simulink model "shoulder_simulink"  (R2024b)
settings: Solver=VariableStepAuto  StartTime=0.0  StopTime=10  FixedStep=0.02  MaxStep=5e-4  RelTol=1e-3  AbsTol=1e-3  EnableMultiTasking=on
InitFcn:
  | main;
values from neighbouring files (symbols this model uses):
  activ = zeros(35,1)    [main_quat.m]
  fmax = sym('fmax', [length(muscles) 1])    [muscle_derivation.m]
  fmax_optim = x_new(11:11+nmus-1)    [SteadyPosOptEul.m]    (also in SteadyPosOptQuat.m = x_new(qn+1:qn+1+nmus-1); steady_position_optimization.m)
  initCond_optim = [x_new(1:10);zeros(10,1)]    [SteadyPosOptEul.m]
  initEul = params.InitPosOptEul.initCondEul    [main.m]
  initQuat = params.InitPosOptEul.initCondQuat    [main.m]
  lceopt = sym('lceopt', [length(muscles) 1])    [muscle_derivation.m]
  lceopt_optim = x_new(11+nmus:end-1)    [SteadyPosOptEul.m]    (also in SteadyPosOptQuat.m = x_new(qn+1+nmus:end); steady_position_optimization.m = x_new(11+nmus:end))
  lslack = sym('lslack', [length(muscles) 1])    [muscle_derivation.m]
  lslack_optim = lslack_vec    [SteadyPosOptEul.m]    (also in SteadyPosOptQuat.m; steady_position_optimization.m)
  m = [2.0519,0.5464,0.5464,0.525]    [data.m]
  model = das3_readosim(osim_file,[motion_path,'\',mydir '\' musclepoly_file])    [create_motion_files.m]    (also in das3_polynomials.m = das3_readosim(osimfile); data_model_eul.mat = ; data_model_mod.mat = ; main.m = data.params.model)
  params = data.params    [SteadyPosOptEul.m]    (also in data_model.mat = ; main.m)
  s = fx.getSize()    [das3_readosim.m]
undefined symbols (not defined in the file or in its folder): h_ej, initCondOptim, initSimScape, phi_0, r_0, r_10, r_20, r_ej, T_d, X, Y, Z
libraries: sm_lib x80, nesl_utility x39
(part 3 of 3)

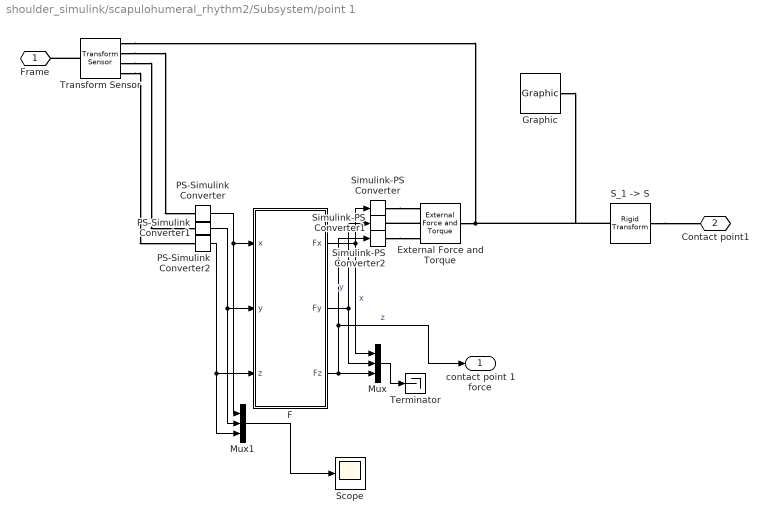
== system shoulder_simulink/scapulohumeral_rhythm2/Subsystem/point 1 ==
  External Force and Torque : sm_lib/Forces and Torques/External Force and Torque  EnableForceX=on  EnableForceY=on  EnableForceZ=on  EnableForce=off  ForceResolutionFrame=World  EnableTorqueX=off  EnableTorqueY=off  EnableTorqueZ=off  EnableTorque=off  TorqueResolutionFrame=AttachedFrame
  F : MATLAB Function  TreatAsAtomicUnit=on
  Graphic : sm_lib/Body Elements/Graphic  GraphicType=Marker  MarkerShape=Sphere  MarkerSize=10  GraphicVisPropType=SimpleVisualProperties  GraphicDiffuseColor=[0 1 0]  GraphicOpacity=1.0  GraphicSpecularColor=[0.5 0.5 0.5 1.0]  GraphicAmbientColor=[0.15 0.15 0.15 1.0]  GraphicEmissiveColor=[0.0 0.0 0.0 1.0]  GraphicShininess=75
  Mux : Mux  Inputs=3
  Mux1 : Mux  Inputs=3
  PS-Simulink Converter : nesl_utility/PS-Simulink Converter  PhysicalDomain=network_engine_domain  SubClassName=ps_output  LeftPortType=input  RightPortType=output  PseudoPeriodic=off  Frequencies=[]  VectorFormat=inherit  Unit=inherit  AffineConversion=off
  PS-Simulink Converter1 : nesl_utility/PS-Simulink Converter  PhysicalDomain=network_engine_domain  SubClassName=ps_output  LeftPortType=input  RightPortType=output  PseudoPeriodic=off  Frequencies=[]  VectorFormat=inherit  Unit=inherit  AffineConversion=off
  PS-Simulink Converter2 : nesl_utility/PS-Simulink Converter  PhysicalDomain=network_engine_domain  SubClassName=ps_output  LeftPortType=input  RightPortType=output  PseudoPeriodic=off  Frequencies=[]  VectorFormat=inherit  Unit=inherit  AffineConversion=off
  "S_1 -> S" : sm_lib/Frames and Transforms/Rigid Transform  RotationMethod=None  FollAlignAxisA=+X  BaseAlignAxisA=+Y  FollAlignAxisB=+Y  BaseAlignAxisB=+Z  RotationStandardAxis=+Z  RotationAngle=0.0  RotationAngleUnits=deg  RotationArbitraryAxis=[0 0 1]  RotationSequenceAxes=FollowerAxes  RotationSequence=XYX  RotationSequenceAngles=[0 0 0]  RotationSequenceAnglesUnits=deg  RotationMatrix=[1 0 0; 0 1 0; 0 0 1]  Quaternion=[1 0 0 0]  TranslationMethod=Cartesian  TranslationCartesianOffset=model.contTS  TranslationCartesianOffsetUnits=m  TranslationStandardAxis=+Z  TranslationStandardOffset=0  TranslationStandardOffsetUnits=m  TranslationROffset=0  TranslationROffsetUnits=m  TranslationThetaOffset=0  TranslationThetaOffsetUnits=deg  TranslationZOffset=0  TranslationZOffsetUnits=m
  Scope : Scope
  Simulink-PS Converter : nesl_utility/Simulink-PS Converter  PhysicalDomain=network_engine_domain  SubClassName=ps_input  LeftPortType=input  RightPortType=output  PseudoPeriodic=off  Frequencies=[]  NoiseDistribution=none  NoiseParameters=[]  Unit=1  AffineConversion=off  FilteringAndDerivatives=provide  SimscapeFilterOrder=1  InputFilterTimeConstant=0.001  UdotUserProvided=0
  Simulink-PS Converter1 : nesl_utility/Simulink-PS Converter  PhysicalDomain=network_engine_domain  SubClassName=ps_input  LeftPortType=input  RightPortType=output  PseudoPeriodic=off  Frequencies=[]  NoiseDistribution=none  NoiseParameters=[]  Unit=1  AffineConversion=off  FilteringAndDerivatives=provide  SimscapeFilterOrder=1  InputFilterTimeConstant=0.001  UdotUserProvided=0
  Simulink-PS Converter2 : nesl_utility/Simulink-PS Converter  PhysicalDomain=network_engine_domain  SubClassName=ps_input  LeftPortType=input  RightPortType=output  PseudoPeriodic=off  Frequencies=[]  NoiseDistribution=none  NoiseParameters=[]  Unit=1  AffineConversion=off  FilteringAndDerivatives=provide  SimscapeFilterOrder=1  InputFilterTimeConstant=0.001  UdotUserProvided=0
  Terminator : Terminator
  Transform Sensor : sm_lib/Frames and Transforms/Transform Sensor  MeasurementFrame=World  RotationSequence=XYX  SenseAngle=off  SenseAxis=off  SenseQ=off  SenseR=off  SenseRotationSequence=off  SenseOmegaX=off  SenseOmegaY=off  SenseOmegaZ=off  SenseOmega=off  SenseQDot=off  SenseRDot=off  SenseRotationSequenceDot=off  SenseAlphaX=off  SenseAlphaY=off  SenseAlphaZ=off  SenseAlpha=off  SenseQDDot=off  SenseRDDot=off  SenseX=on  SenseY=on  SenseZ=on  SenseXYZ=off  SenseRad=off  SenseAzim=off  SenseDist=off  SenseInc=off  SenseXDot=off  SenseYDot=off  SenseZDot=off  SenseXYZDot=off  SenseRadDot=off  SenseAzimDot=off  SenseDistDot=off  SenseIncDot=off  SenseXDDot=off  SenseYDDot=off  SenseZDDot=off  SenseXYZDDot=off  SenseRadDDot=off  SenseAzimDDot=off  SenseDistDDot=off  SenseIncDDot=off
  Frame : PMIOPort  Side=Left
  Contact point1 : PMIOPort  Port=2  Side=Right
  contact point 1 force : Outport
  wires:
  PS-Simulink Converter2/1 -> Mux1/3, F/3(z)
  F/3(Fz) -> contact point 1 force/1, Simulink-PS Converter2/1, Mux/3  "z"
  PS-Simulink Converter1/1 -> Mux1/2, F/2(y)
  F/1(Fx) -> Simulink-PS Converter/1, Mux/1  "x"
  F/2(Fy) -> Simulink-PS Converter1/1, Mux/2  "y"
  PS-Simulink Converter/1 -> Mux1/1, F/1(x)
  Mux1/1 -> Scope/1
  Mux/1 -> Terminator/1
  connections:
  External Force and Torque/LConn2 -- Simulink-PS Converter1/RConn1
  Transform Sensor/RConn4 -- PS-Simulink Converter2/LConn1
  Transform Sensor/RConn2 -- PS-Simulink Converter/LConn1
  Transform Sensor/LConn1 -- Frame/RConn1
  Simulink-PS Converter/RConn1 -- External Force and Torque/LConn1
  Transform Sensor/RConn3 -- PS-Simulink Converter1/LConn1
  Simulink-PS Converter2/RConn1 -- External Force and Torque/LConn3
  External Force and Torque/RConn1 -- Graphic/RConn1 -- "S_1 -> S"/RConn1 -- Transform Sensor/RConn1
  "S_1 -> S"/LConn1 -- Contact point1/RConn1

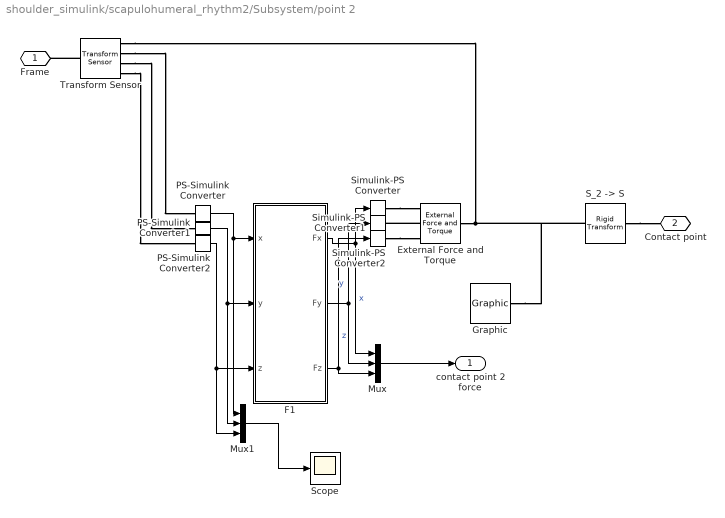
== system shoulder_simulink/scapulohumeral_rhythm2/Subsystem/point 2 ==
  External Force and Torque : sm_lib/Forces and Torques/External Force and Torque  EnableForceX=on  EnableForceY=on  EnableForceZ=on  EnableForce=off  ForceResolutionFrame=World  EnableTorqueX=off  EnableTorqueY=off  EnableTorqueZ=off  EnableTorque=off  TorqueResolutionFrame=AttachedFrame
  F1 : MATLAB Function  TreatAsAtomicUnit=on
  Graphic : sm_lib/Body Elements/Graphic  GraphicType=Marker  MarkerShape=Sphere  MarkerSize=10  GraphicVisPropType=SimpleVisualProperties  GraphicDiffuseColor=[0 1 0]  GraphicOpacity=1.0  GraphicSpecularColor=[0.5 0.5 0.5 1.0]  GraphicAmbientColor=[0.15 0.15 0.15 1.0]  GraphicEmissiveColor=[0.0 0.0 0.0 1.0]  GraphicShininess=75
  Mux : Mux  Inputs=3
  Mux1 : Mux  Inputs=3
  PS-Simulink Converter : nesl_utility/PS-Simulink Converter  PhysicalDomain=network_engine_domain  SubClassName=ps_output  LeftPortType=input  RightPortType=output  PseudoPeriodic=off  Frequencies=[]  VectorFormat=inherit  Unit=inherit  AffineConversion=off
  PS-Simulink Converter1 : nesl_utility/PS-Simulink Converter  PhysicalDomain=network_engine_domain  SubClassName=ps_output  LeftPortType=input  RightPortType=output  PseudoPeriodic=off  Frequencies=[]  VectorFormat=inherit  Unit=inherit  AffineConversion=off
  PS-Simulink Converter2 : nesl_utility/PS-Simulink Converter  PhysicalDomain=network_engine_domain  SubClassName=ps_output  LeftPortType=input  RightPortType=output  PseudoPeriodic=off  Frequencies=[]  VectorFormat=inherit  Unit=inherit  AffineConversion=off
  "S_2 -> S" : sm_lib/Frames and Transforms/Rigid Transform  RotationMethod=None  FollAlignAxisA=+X  BaseAlignAxisA=+Y  FollAlignAxisB=+Y  BaseAlignAxisB=+Z  RotationStandardAxis=+Z  RotationAngle=0.0  RotationAngleUnits=deg  RotationArbitraryAxis=[0 0 1]  RotationSequenceAxes=FollowerAxes  RotationSequence=XYX  RotationSequenceAngles=[0 0 0]  RotationSequenceAnglesUnits=deg  RotationMatrix=[1 0 0; 0 1 0; 0 0 1]  Quaternion=[1 0 0 0]  TranslationMethod=Cartesian  TranslationCartesianOffset=model.contAI  TranslationCartesianOffsetUnits=m  TranslationStandardAxis=+Z  TranslationStandardOffset=0  TranslationStandardOffsetUnits=m  TranslationROffset=0  TranslationROffsetUnits=m  TranslationThetaOffset=0  TranslationThetaOffsetUnits=deg  TranslationZOffset=0  TranslationZOffsetUnits=m
  Scope : Scope
  Simulink-PS Converter : nesl_utility/Simulink-PS Converter  PhysicalDomain=network_engine_domain  SubClassName=ps_input  LeftPortType=input  RightPortType=output  PseudoPeriodic=off  Frequencies=[]  NoiseDistribution=none  NoiseParameters=[]  Unit=1  AffineConversion=off  FilteringAndDerivatives=provide  SimscapeFilterOrder=1  InputFilterTimeConstant=0.001  UdotUserProvided=0
  Simulink-PS Converter1 : nesl_utility/Simulink-PS Converter  PhysicalDomain=network_engine_domain  SubClassName=ps_input  LeftPortType=input  RightPortType=output  PseudoPeriodic=off  Frequencies=[]  NoiseDistribution=none  NoiseParameters=[]  Unit=1  AffineConversion=off  FilteringAndDerivatives=provide  SimscapeFilterOrder=1  InputFilterTimeConstant=0.001  UdotUserProvided=0
  Simulink-PS Converter2 : nesl_utility/Simulink-PS Converter  PhysicalDomain=network_engine_domain  SubClassName=ps_input  LeftPortType=input  RightPortType=output  PseudoPeriodic=off  Frequencies=[]  NoiseDistribution=none  NoiseParameters=[]  Unit=1  AffineConversion=off  FilteringAndDerivatives=provide  SimscapeFilterOrder=1  InputFilterTimeConstant=0.001  UdotUserProvided=0
  Transform Sensor : sm_lib/Frames and Transforms/Transform Sensor  MeasurementFrame=World  RotationSequence=XYX  SenseAngle=off  SenseAxis=off  SenseQ=off  SenseR=off  SenseRotationSequence=off  SenseOmegaX=off  SenseOmegaY=off  SenseOmegaZ=off  SenseOmega=off  SenseQDot=off  SenseRDot=off  SenseRotationSequenceDot=off  SenseAlphaX=off  SenseAlphaY=off  SenseAlphaZ=off  SenseAlpha=off  SenseQDDot=off  SenseRDDot=off  SenseX=on  SenseY=on  SenseZ=on  SenseXYZ=off  SenseRad=off  SenseAzim=off  SenseDist=off  SenseInc=off  SenseXDot=off  SenseYDot=off  SenseZDot=off  SenseXYZDot=off  SenseRadDot=off  SenseAzimDot=off  SenseDistDot=off  SenseIncDot=off  SenseXDDot=off  SenseYDDot=off  SenseZDDot=off  SenseXYZDDot=off  SenseRadDDot=off  SenseAzimDDot=off  SenseDistDDot=off  SenseIncDDot=off
  Frame : PMIOPort  Side=Left
  Contact point : PMIOPort  Port=2  Side=Right
  contact point 2 force : Outport
  wires:
  PS-Simulink Converter/1 -> F1/1(x), Mux1/1
  F1/2(Fy) -> Simulink-PS Converter1/1, Mux/2  "y"
  F1/1(Fx) -> Mux/1, Simulink-PS Converter/1  "x"
  PS-Simulink Converter1/1 -> F1/2(y), Mux1/2
  Mux/1 -> contact point 2 force/1
  F1/3(Fz) -> Simulink-PS Converter2/1, Mux/3  "z"
  PS-Simulink Converter2/1 -> F1/3(z), Mux1/3
  Mux1/1 -> Scope/1
  connections:
  Transform Sensor/RConn1 -- Graphic/RConn1 -- "S_2 -> S"/RConn1 -- External Force and Torque/RConn1
  Simulink-PS Converter2/RConn1 -- External Force and Torque/LConn3
  Transform Sensor/RConn3 -- PS-Simulink Converter1/LConn1
  Simulink-PS Converter/RConn1 -- External Force and Torque/LConn1
  Transform Sensor/LConn1 -- Frame/RConn1
  Transform Sensor/RConn2 -- PS-Simulink Converter/LConn1
  Transform Sensor/RConn4 -- PS-Simulink Converter2/LConn1
  External Force and Torque/LConn2 -- Simulink-PS Converter1/RConn1
  "S_2 -> S"/LConn1 -- Contact point/RConn1

== system shoulder_simulink/scapulohumeral_rhythm2/2_points_contact/tools/cartensian_X ==
  Mux : Mux  Inputs=3
  PS-Simulink Converter : nesl_utility/PS-Simulink Converter  PhysicalDomain=network_engine_domain  SubClassName=ps_output  LeftPortType=input  RightPortType=output  PseudoPeriodic=off  Frequencies=[]  VectorFormat=inherit  Unit=inherit  AffineConversion=off
  PS-Simulink Converter1 : nesl_utility/PS-Simulink Converter  PhysicalDomain=network_engine_domain  SubClassName=ps_output  LeftPortType=input  RightPortType=output  PseudoPeriodic=off  Frequencies=[]  VectorFormat=inherit  Unit=inherit  AffineConversion=off
  PS-Simulink Converter2 : nesl_utility/PS-Simulink Converter  PhysicalDomain=network_engine_domain  SubClassName=ps_output  LeftPortType=input  RightPortType=output  PseudoPeriodic=off  Frequencies=[]  VectorFormat=inherit  Unit=inherit  AffineConversion=off
  To Workspace : ToWorkspace  VariableName=X  SampleTime=-1
  Transform Sensor : sm_lib/Frames and Transforms/Transform Sensor  MeasurementFrame=World  RotationSequence=XYX  SenseAngle=off  SenseAxis=off  SenseQ=off  SenseR=off  SenseRotationSequence=off  SenseOmegaX=off  SenseOmegaY=off  SenseOmegaZ=off  SenseOmega=off  SenseQDot=off  SenseRDot=off  SenseRotationSequenceDot=off  SenseAlphaX=off  SenseAlphaY=off  SenseAlphaZ=off  SenseAlpha=off  SenseQDDot=off  SenseRDDot=off  SenseX=on  SenseY=on  SenseZ=on  SenseXYZ=off  SenseRad=off  SenseAzim=off  SenseDist=off  SenseInc=off  SenseXDot=off  SenseYDot=off  SenseZDot=off  SenseXYZDot=off  SenseRadDot=off  SenseAzimDot=off  SenseDistDot=off  SenseIncDot=off  SenseXDDot=off  SenseYDDot=off  SenseZDDot=off  SenseXYZDDot=off  SenseRadDDot=off  SenseAzimDDot=off  SenseDistDDot=off  SenseIncDDot=off
  World Frame : sm_lib/Frames and Transforms/World Frame
  X : PMIOPort  Side=Left
  wires:
  PS-Simulink Converter/1 -> Mux/1
  Mux/1 -> To Workspace/1
  PS-Simulink Converter1/1 -> Mux/2
  PS-Simulink Converter2/1 -> Mux/3
  connections:
  Transform Sensor/RConn4 -- PS-Simulink Converter2/LConn1
  Transform Sensor/RConn2 -- PS-Simulink Converter/LConn1
  PS-Simulink Converter1/LConn1 -- Transform Sensor/RConn3
  Transform Sensor/RConn1 -- X/RConn1
  World Frame/RConn1 -- Transform Sensor/LConn1

== matlab function shoulder_simulink/Subsystem3/MATLAB Function ==
  data: Q input; y output; dQ input
function y = fcn(Q,dQ)

y = 2*G(Q)*dQ;

end

function res = G(Q)
Q0 = Q(1);
Q1 = Q(2);
Q2 = Q(3);
Q3 = Q(4);
res = [-Q1, Q0, Q3, -Q2;
        -Q2,-Q3, Q0, Q1;
        -Q3, Q2, -Q1, Q0];
end

== matlab function shoulder_simulink/eoms sympy3 ==
  data: t input; x input; act input; model parameter; lslack_optim parameter; lceopt_optim parameter; y output; fmax_optim parameter
function y = fcn(t,x,act,model,lslack_optim, lceopt_optim, fmax_optim)
y = zeros(20,1);
MM = mm_py_ulna_InOutCont(t,x,model);
FO = fo_py_ulna_InOutCont(t,x,model);
FE_muscles = f_muscles_ulna(t,x(1:10),act,fmax_optim,lceopt_optim,lslack_optim);
y = MM\(FO+FE_muscles);

== matlab function shoulder_simulink/scapulohumeral_rhythm2/1_point_contact/phi = fcn(h) ==
  data: h input; phi output; h_ej parameter; r_ej parameter
function phi = fcn(h,h_ej,r_ej)

phi = atan(-(r_ej*h)/(h_ej^2*sqrt(1-h^2/h_ej^2)));

== matlab function shoulder_simulink/scapulohumeral_rhythm2/1_point_contact/r = fcn(h) ==
  data: h input; r output; h_ej parameter; r_ej parameter
function r = fcn(h,h_ej,r_ej)

r = sqrt((r_ej^2)*(1-h^2/h_ej^2));

== matlab function shoulder_simulink/scapulohumeral_rhythm2/2_points_contact/ellipsoidal_joint_1/r = fcn(h) ==
  data: h input; r output; h_ej parameter; r_ej parameter
function r = fcn(h,h_ej,r_ej)

r = sqrt((r_ej^2)*(1-h^2/h_ej^2));

== matlab function shoulder_simulink/scapulohumeral_rhythm2/2_points_contact/ellipsoidal_joint_2/r = fcn(h) ==
  data: h input; r output; h_ej parameter; r_ej parameter
function r = fcn(h,h_ej,r_ej)

r = sqrt((r_ej^2)*(1-h^2/h_ej^2));

== matlab function shoulder_simulink/scapulohumeral_rhythm2/Subsystem/point 1/F ==
  data: x input; Fx output; y input; z input; Fy output; Fz output; model parameter
function [Fx,Fy,Fz]= fcn(x,y,z,model)

f_in = ((x-model.elips_trans(1))/(model.first_elips_scale*model.elips_dim(1)))^2+((y-model.elips_trans(2))/(model.first_elips_scale*model.elips_dim(2)))^2+((z-model.elips_trans(3))/(model.first_elips_scale*model.elips_dim(3)))^2-1;
f_out = ((x-model.elips_trans(1))/(model.second_elips_scale*model.elips_dim(1)))^2+((y-model.elips_trans(2))/(model.second_elips_scale*model.elips_dim(2)))^2+((z-model.elips_trans(3))/(model.second_elips_scale*model.elips_dim(3)))^2-1;
F_in = 1/2*(f_in-sqrt(f_in^2+model.eps_in^2));
F_out = 1/2*(f_out+sqrt(f_out^2+model.eps_out^2));

Fx = -(model.k_contact_in*F_in+model.k_contact_out*F_out)*(x-model.elips_trans(1))*(model.elips_dim(1)^2+model.elips_dim(2)^2+model.elips_dim(3)^2)/(model.elips_dim(1)^2);
Fy = -(model.k_contact_in*F_in+model.k_contact_out*F_out)*(y-model.elips_trans(2))*(model.elips_dim(1)^2+model.elips_dim(2)^2+model.elips_dim(3)^2)/(model.elips_dim(2)^2);
Fz = -(model.k_contact_in*F_in+model.k_contact_out*F_out)*(z-model.elips_trans(3))*(model.elips_dim(1)^2+model.elips_dim(2)^2+model.elips_dim(3)^2)/(model.elips_dim(3)^2);

%% 2D
% 
% f = ((x-mx)/model.elips_dim(1))^2+((z-mz)/model.elips_dim(3))^2-1;
% F = 1/2*(f-sqrt(f^2+eps^2));
% 
% Fx = -k*(x-mx)*(model.elips_dim(1)^2+model.elips_dim(2)^2)/(model.elips_dim(1)^2)*F;
% Fy = -k*(y-my)*(model.elips_dim(1)^2+model.elips_dim(2)^2)/(model.elips_dim(2)^2)*F;
% Fz = -k*(z-mz)*(model.elips_dim(1)^2+model.elips_dim(2)^2)/(model.elips_dim(3)^2)*F;

== matlab function shoulder_simulink/scapulohumeral_rhythm2/Subsystem/point 2/F1 ==
  data: x input; Fx output; y input; z input; Fy output; Fz output; model parameter
function [Fx,Fy,Fz]= fcn(x,y,z,model)

f_in = ((x-model.elips_trans(1))/(model.first_elips_scale*model.elips_dim(1)))^2+((y-model.elips_trans(2))/(model.first_elips_scale*model.elips_dim(2)))^2+((z-model.elips_trans(3))/(model.first_elips_scale*model.elips_dim(3)))^2-1;
f_out = ((x-model.elips_trans(1))/(model.second_elips_scale*model.elips_dim(1)))^2+((y-model.elips_trans(2))/(model.second_elips_scale*model.elips_dim(2)))^2+((z-model.elips_trans(3))/(model.second_elips_scale*model.elips_dim(3)))^2-1;
F_in = 1/2*(f_in-sqrt(f_in^2+model.eps_in^2));
F_out = 1/2*(f_out+sqrt(f_out^2+model.eps_out^2));

Fx = -(model.k_contact_in*F_in+model.k_contact_out*F_out)*(x-model.elips_trans(1))*(model.elips_dim(1)^2+model.elips_dim(2)^2+model.elips_dim(3)^2)/(model.elips_dim(1)^2);
Fy = -(model.k_contact_in*F_in+model.k_contact_out*F_out)*(y-model.elips_trans(2))*(model.elips_dim(1)^2+model.elips_dim(2)^2+model.elips_dim(3)^2)/(model.elips_dim(2)^2);
Fz = -(model.k_contact_in*F_in+model.k_contact_out*F_out)*(z-model.elips_trans(3))*(model.elips_dim(1)^2+model.elips_dim(2)^2+model.elips_dim(3)^2)/(model.elips_dim(3)^2);

%% 2D
% 
% f = ((x-mx)/model.elips_dim(1))^2+((z-mz)/model.elips_dim(3))^2-1;
% F = 1/2*(f-sqrt(f^2+eps^2));
% 
% Fx = -k*(x-mx)*(model.elips_dim(1)^2+model.elips_dim(2)^2)/(model.elips_dim(1)^2)*F;
% Fy = -k*(y-my)*(model.elips_dim(1)^2+model.elips_dim(2)^2)/(model.elips_dim(2)^2)*F;
% Fz = -k*(z-mz)*(model.elips_dim(1)^2+model.elips_dim(2)^2)/(model.elips_dim(3)^2)*F;

== matlab function shoulder_simulink/EUL ==
  data: x input; model parameter; y output; qSC output; qAC output; qGH output; qulna output; params parameter; act input; qradius output
function [y,qSC,qAC,qGH,qulna,qradius] = fcn(x,model,params,act)
%, sh_e, T_el, eps, k_contact, cont_P, akt, force, l0m
qSC = x(1:3);
qAC = x(4:6);
qGH = x(7:9);
qulna = x(10);
qradius = x(11);
t = 0;

% fmax = params.InitPosOptQuat.fmax;
% lceopt = params.InitPosOptQuat.lceopt;
% lslack = params.InitPosOptQuat.lslack;

first_elips_scale = model.first_elips_scale;
y = zeros(22,1);
MM = mm_eul(t,x(1:11),x(12:22),model,[first_elips_scale]);
FO = fo_eul(t,x(1:11),x(12:22),model,[first_elips_scale]);
% TE_conoid = [zeros(10,1);TE_conoid_eul(t,x,0,0,0)'];
% FE = TE_full_eul(t,[zeros(3,1);x(1:10);0],act,fmax,lceopt,lslack);
y = MM\(FO);

== matlab function shoulder_simulink/QUAT ==
  data: x input; y output; params parameter; q1s output; q2s output; q3s output; q4s output; model parameter; q5 output; act input
function [y,q1s,q2s,q3s,q4s,q5] = fcn(x,params,model,act)
y = zeros(25,1);
q1 = x(1:4);
q2 = x(5:8);
q3 = x(9:12);
q4 = x(13);
q5 = x(14);
q1new = q1/norm(q1);
q2new = q2/norm(q2);
q3new = q3/norm(q2);
u = x(15:end);
t = 0;
q1s = q1new;
q2s = q2new;
q3s = q3new;
q4s = q4;

% fmax = params.InitPosOptQuat.fmax;
% lceopt = params.InitPosOptQuat.lceopt;
% lslack = params.InitPosOptQuat.lslack;
parameters = [model.first_elips_scale];

mm = mm_quat(t,[q1new;q2new;q3new;x(13);x(14)],u,model,parameters);
fo = fo_quat(t,[q1new;q2new;q3new;x(13);x(14)],u,model,parameters);
% fe = TE_full_quat(t,[zeros(4,1);[q1new;q2new;q3new;q4];0],act,fmax,lceopt,lslack);
y = mm\(fo);

end

== matlab function shoulder_simulink/MATLAB Function1 ==
  data: y output; x input; act input; lslack_optim parameter; lceopt_optim parameter; fmax_optim parameter
function y = fcn(x,act, lslack_optim, lceopt_optim, fmax_optim)
t = 0;
y = mus_forces_ulna(t,x,act,fmax_optim,lceopt_optim,lslack_optim);

== matlab function shoulder_simulink/MATLAB Function ==
  data: u input; y output; lceopt_optim parameter; lslack_optim parameter
function y = fcn(u,lceopt_optim,lslack_optim)
t = 0;
lm = mus_lengths_ulna(t,u)';
% y = zeros(35,1);
y = (lm-lslack_optim) ./ lceopt_optim;

== matlab function shoulder_simulink/MATLAB Function3 ==
  data: t input; act output
function act = fcn(t)
% t_end = 2;
act = zeros(137,1);
% act(1:11) = 0.25*t/t_end;
% act(45:47) = 0.6*t/t_end;

== matlab function shoulder_simulink/MATLAB Function5 ==
  data: t input; act output
function act = fcn(t)
% t_end = 2;
act = zeros(137,1);
% act(1:11) = 0.02 + 0.15*t/t_end;
% act(45:47) = 0.1 + 0.5*t/t_end;

== matlab function shoulder_simulink/Subsystem/MATLAB Function ==
  data: l input; F output; d output
function [F,d] = fcn(l)
lopt = 0.05;
k = 80000;
eps = 1.00e-05;
d = l-lopt;
F = -k/2*(d+sqrt(d^2+eps));

== matlab function shoulder_simulink/eoms sympy2 ==
  data: t input; x input; act input; model parameter; y output; fmax parameter; lceopt parameter; lslack parameter
function y = fcn(t,x,act,model,fmax, lceopt, lslack)
%, sh_e, T_el, eps, k_contact, cont_P, akt, force, l0m
y = zeros(22,1);
MM = mm_py_full(t,x,model);
FO = fo_py_full(t,x,model);
FE_muscles = f_muscles(t,x(1:11),act,fmax,lceopt,lslack);
% FE = fe(t,[x(1:6)',x(7:12)'],force,l0m,akt');
y = MM\(FO+FE_muscles);
